simulink model "LQR_Simulink"  (R2023b)
settings: Solver=VariableStepAuto  StartTime=0.0  StopTime=10  RelTol=1e-10
undefined symbols (not defined in the file): K, x_e
settings Model: Creator=franc  LastModifiedBy=franc

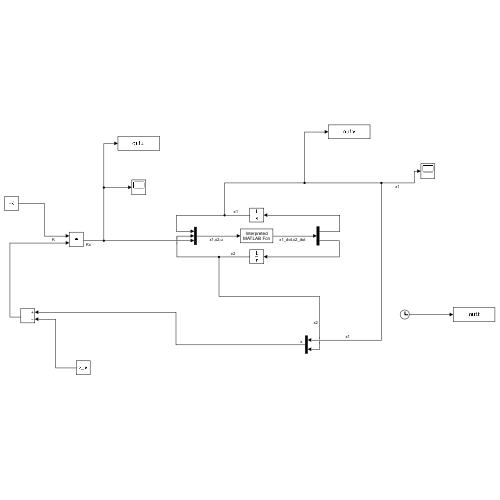
[thumbnail: Simulink's stored preview of the top-level diagram]
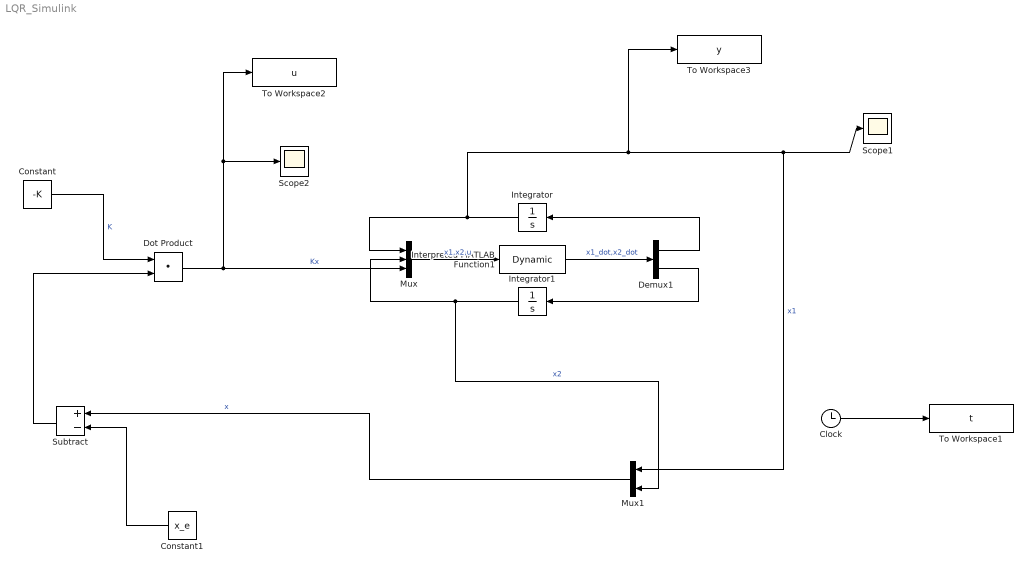
== system LQR_Simulink ==
  Clock : Clock
  Constant : Constant  Value=-K
  Constant1 : Constant  Value=x_e
  Demux1 : Demux  Outputs=2
  Dot Product : DotProduct  OutDataTypeStr=Inherit: Inherit via internal rule
  Integrator : Integrator
  Integrator1 : Integrator
  Interpreted MATLAB Function1 : MATLABFcn  MATLABFcn=Dynamic  OutputDimensions=2
  Mux : Mux  Inputs=3
  Mux1 : Mux  Inputs=2
  Scope1 : Scope
  Scope2 : Scope
  Subtract : Sum  Inputs=+-
  To Workspace1 : ToWorkspace  VariableName=t  SampleTime=-1
  To Workspace2 : ToWorkspace  VariableName=u  SampleTime=-1
  To Workspace3 : ToWorkspace  VariableName=y  SampleTime=-1
  wires:
  Interpreted MATLAB Function1/1 -> Demux1/1  "x1_dot,x2_dot"
  Constant/1 -> Dot Product/1  "K"
  Demux1/2 -> Integrator1/1
  Demux1/1 -> Integrator/1
  Mux/1 -> Interpreted MATLAB Function1/1  "x1,x2,u"
  Integrator/1 -> To Workspace3/1, Mux1/1, Scope1/1, Mux/1  "x1"
  Integrator1/1 -> Mux1/2, Mux/2  "x2"
  Clock/1 -> To Workspace1/1
  Dot Product/1 -> To Workspace2/1, Scope2/1, Mux/3  "Kx"
  Mux1/1 -> Subtract/1  "x"
  Constant1/1 -> Subtract/2
  Subtract/1 -> Dot Product/2
